simulink model "Lab_7_task_1_4"  (R2020b)
settings: Solver=ode113  StartTime=0.0  StopTime=T  RelTol=1e-13
values from neighbouring files (symbols this model uses):
  a = 8.6251e+06    (= 8625100)    [Quaternions_method_parameters.m]    (also in car2kep.m = -(mu/(2*E)))
  e = norm(e)    [Lab_7_task_1_4_parameters.m]    (also in Lab_7_task_5_parameters.m; Quaternions_method_parameters.m = 0.1195; car2kep.m = 1/mu * [((v_norm)^2 - (mu/r_norm)).*r - (dot(r, v).*v)])
  G = 6.67259e-11    [Lab_7_task_1_4_parameters.m]    (also in Lab_7_task_5_parameters.m; Quaternions_method_parameters.m)
  i = acos(h_z/h_norm)    [car2kep.m]
  I_x = 0.04    [Lab_7_task_1_4_parameters.m]    (also in Lab_7_task_5_parameters.m)
  I_y = 0.06    [Lab_7_task_1_4_parameters.m]    (also in Lab_7_task_5_parameters.m)
  I_z = 0.08    [Lab_7_task_1_4_parameters.m]    (also in Lab_7_task_5_parameters.m)
  m_t = 5.9726*10^24    (= 5.9726e+24)    [Lab_7_task_1_4_parameters.m]    (also in Lab_7_task_5_parameters.m)
  th_0 = 0    [Lab_7_task_1_4_parameters.m]    (also in Lab_7_task_5_parameters.m)
  w_x_0 = 1e-6    (= 1e-06)    [Lab_7_task_1_4_parameters.m]    (also in Lab_7_task_5_parameters.m)
  w_y_0 = 1e-6    (= 1e-06)    [Lab_7_task_1_4_parameters.m]    (also in Lab_7_task_5_parameters.m)
  w_z_0 = n_S    [Lab_7_task_1_4_parameters.m]    (also in Lab_7_task_5_parameters.m)
undefined symbols (not defined in the file or in its folder): magnitude
libraries: robotcorelib x2
settings Model: Creator=39342  LastModifiedBy=39342

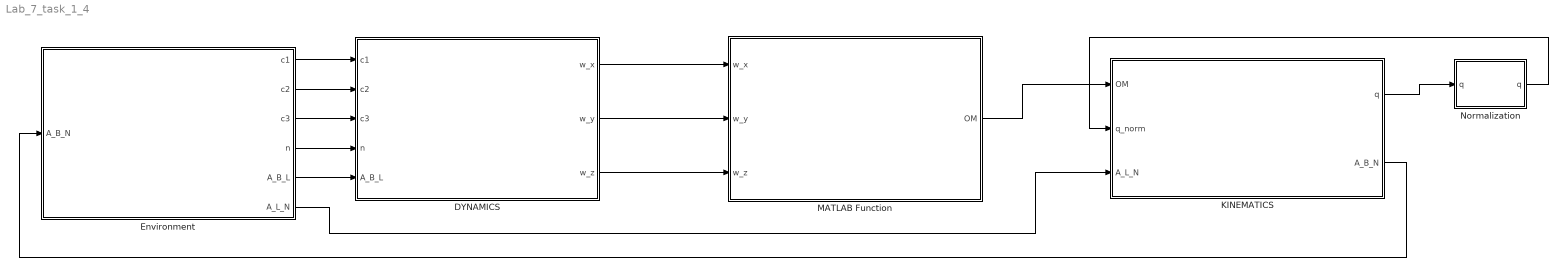
== system Lab_7_task_1_4 ==
  DYNAMICS : Subsystem
  Environment : Subsystem
  KINEMATICS : Subsystem
  MATLAB Function : MATLAB Function  TreatAsAtomicUnit=on
  Normalization : MATLAB Function  TreatAsAtomicUnit=on
  wires:
  Environment/3(c3) -> DYNAMICS/3(c3)
  Environment/1(c1) -> DYNAMICS/1(c1)
  DYNAMICS/1(w_x) -> MATLAB Function/1(w_x)
  Environment/2(c2) -> DYNAMICS/2(c2)
  DYNAMICS/2(w_y) -> MATLAB Function/2(w_y)
  DYNAMICS/3(w_z) -> MATLAB Function/3(w_z)
  Normalization/1(q) -> KINEMATICS/2(q_norm)
  MATLAB Function/1(OM) -> KINEMATICS/1(OM)
  KINEMATICS/1(q) -> Normalization/1("q ")
  KINEMATICS/2(A_B_N) -> Environment/1(A_B_N)
  Environment/4(n) -> DYNAMICS/4(n)
  Environment/5(A_B_L) -> DYNAMICS/5(A_B_L)
  Environment/6(A_L_N) -> KINEMATICS/3(A_L_N)

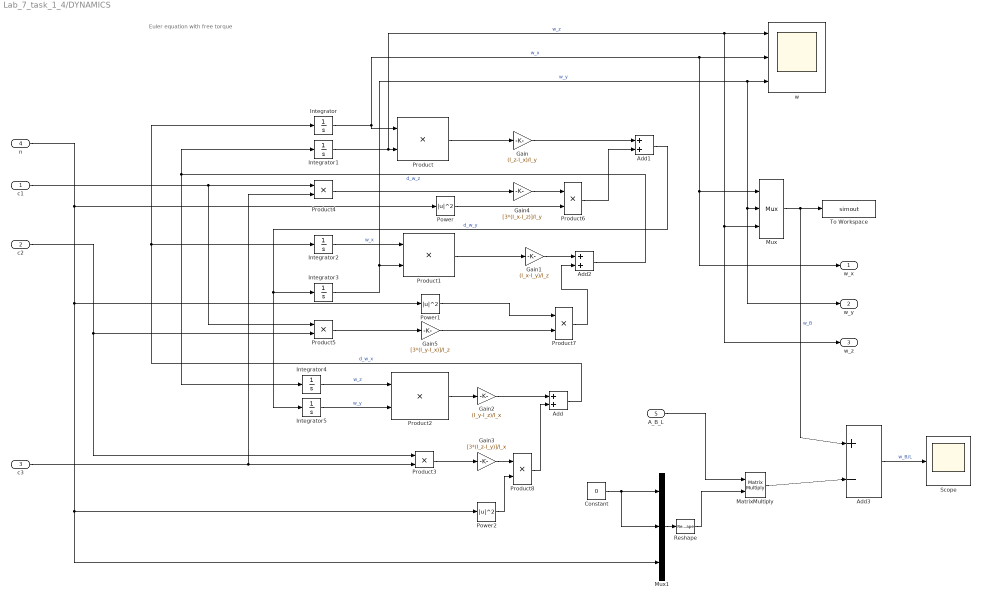
== system Lab_7_task_1_4/DYNAMICS ==
  note: Euler equation with free torque
  c1 : Inport
  c2 : Inport  Port=2
  c3 : Inport  Port=3
  n : Inport  Port=4
  A_B_L : Inport  Port=5
  Add : Sum
  Add1 : Sum
  Add2 : Sum
  Add3 : Sum  Inputs=+|-
  Constant : Constant  Value=0
  Gain : Gain  Gain=(I_z-I_x)/I_y
  Gain1 : Gain  Gain=(I_x-I_y)/I_z
  Gain2 : Gain  Gain=(I_y-I_z)/I_x
  Gain3 : Gain  Gain=[3*(I_z-I_y)]/I_x
  Gain4 : Gain  Gain=[3*(I_x-I_z)]/I_y
  Gain5 : Gain  Gain=[3*(I_y-I_x)]/I_z
  Integrator : Integrator  InitialCondition=w_x_0
  Integrator1 : Integrator  InitialCondition=w_z_0
  Integrator2 : Integrator  InitialCondition=w_x_0
  Integrator3 : Integrator  InitialCondition=w_y_0
  Integrator4 : Integrator  InitialCondition=w_z_0
  Integrator5 : Integrator  InitialCondition=w_y_0
  MatrixMultiply : Product  Multiplication=Matrix(*)
  Mux : Mux  Inputs=3
  Mux1 : Mux  Inputs=3
  Power : Math  Operator=magnitude^2  SaturateOnIntegerOverflow=on
  Power1 : Math  Operator=magnitude^2  SaturateOnIntegerOverflow=on
  Power2 : Math  Operator=magnitude^2  SaturateOnIntegerOverflow=on
  Product{,1..8} (9 alike) : Product
  Reshape : Reshape  OutputDimensionality=Column vector (2-D)
  Scope : Scope
  To Workspace : ToWorkspace  VariableName=simout  SaveFormat=Timeseries  SampleTime=-1
  w : Scope  NumInputPorts=3
  w_x : Outport
  w_y : Outport  Port=2
  w_z : Outport  Port=3
  wires:
  Product1/1 -> Gain1/1
  Integrator/1 -> Product/1, w_x/1, Mux/1, w/2  "w_x"
  Integrator2/1 -> Product1/1  "w_x"
  Mux/1 -> To Workspace/1, Add3/1  "w_B"
  Integrator1/1 -> w/1, w_z/1, Mux/3, Product/2  "w_z"
  Integrator5/1 -> Product2/2  "w_y"
  Integrator4/1 -> Product2/1  "w_z"
  Integrator3/1 -> Product1/2, w/3, w_y/1, Mux/2  "w_y"
  Product/1 -> Gain/1
  Product2/1 -> Gain2/1
  Gain2/1 -> Add/1
  c3/1 -> Product3/2, Product4/2
  c2/1 -> Product5/2, Product3/1
  Product3/1 -> Gain3/1
  Add/1 -> Integrator/1, Integrator2/1  "d_w_x"
  c1/1 -> Product5/1, Product4/1
  Product4/1 -> Gain4/1
  Gain/1 -> Add1/1
  Add1/1 -> Integrator5/1, Integrator3/1  "d_w_y"
  Product5/1 -> Gain5/1
  Gain1/1 -> Add2/1
  Add2/1 -> Integrator4/1, Integrator1/1  "d_w_z"
  Gain4/1 -> Product6/1
  n/1 -> Mux1/3, Power2/1, Power1/1, Power/1
  Power/1 -> Product6/2
  Product6/1 -> Add1/2
  Power1/1 -> Product7/1
  Gain5/1 -> Product7/2
  Product7/1 -> Add2/2
  Power2/1 -> Product8/2
  Gain3/1 -> Product8/1
  Product8/1 -> Add/2
  Constant/1 -> Mux1/2, Mux1/1
  A_B_L/1 -> MatrixMultiply/1
  Mux1/1 -> Reshape/1
  MatrixMultiply/1 -> Add3/2
  Add3/1 -> Scope/1  "w_B/L"
  Reshape/1 -> MatrixMultiply/2

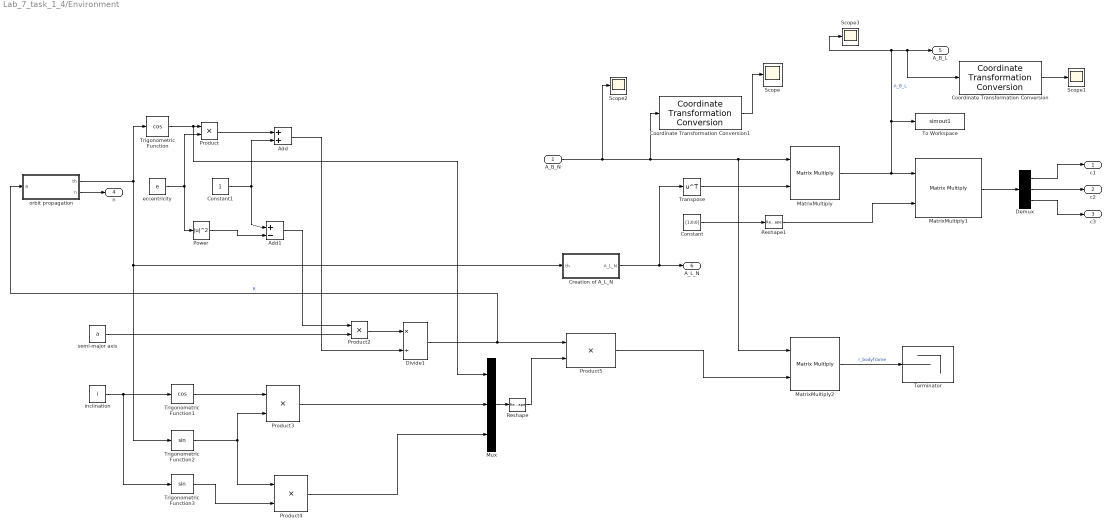
== system Lab_7_task_1_4/Environment ==
  A_B_N : Inport
  Add : Sum
  Add1 : Sum  Inputs=+|-
  Constant : Constant  Value=[1;0;0]
  Constant1 : Constant
  Coordinate Transformation Conversion : robotcorelib/Coordinate Transformation Conversion  InputRepresentation=Rotation Matrix  InputEulerSequence=ZYX  ShowTrVecInputPort=on  OutputRepresentation=Euler Angles  OutputEulerSequence=ZYX  ShowTrVecOutputPort=on  SimulateUsing=Interpreted execution
      settings: SourceProductBaseCode=NV,RO,RR,UV
  Coordinate Transformation Conversion1 : robotcorelib/Coordinate Transformation Conversion  InputRepresentation=Rotation Matrix  InputEulerSequence=ZYX  ShowTrVecInputPort=on  OutputRepresentation=Euler Angles  OutputEulerSequence=ZYX  ShowTrVecOutputPort=on  SimulateUsing=Interpreted execution
      settings: SourceProductBaseCode=NV,RO,RR,UV
  Creation of A_L_N : Subsystem
  Demux : Demux  Outputs=3
  Divide1 : Product  Inputs=*/
  MatrixMultiply : Product  Multiplication=Matrix(*)
  MatrixMultiply1 : Product  Multiplication=Matrix(*)
  MatrixMultiply2 : Product  Multiplication=Matrix(*)
  Mux : Mux  Inputs=3
  Power : Math  Operator=magnitude^2  SaturateOnIntegerOverflow=on
  Product{,2..5} (5 alike) : Product
  Reshape : Reshape  OutputDimensionality=Column vector (2-D)
  Reshape1 : Reshape  OutputDimensionality=Column vector (2-D)
  Scope{,1..3} (4 alike) : Scope
  Terminator : Terminator
  To Workspace : ToWorkspace  VariableName=simout1  SaveFormat=Timeseries  SampleTime=-1
  Transpose : Math  Operator=transpose  SaturateOnIntegerOverflow=on
  Trigonometric Function : Trigonometry  Operator=cos
  Trigonometric Function1 : Trigonometry  Operator=cos
  Trigonometric Function2 : Trigonometry
  Trigonometric Function3 : Trigonometry
  eccentricity : Constant  Value=e
  inclination : Constant  Value=i
  orbit propagation : Subsystem
  semi-major axis : Constant  Value=a
  c1 : Outport
  c2 : Outport  Port=2
  c3 : Outport  Port=3
  n : Outport  Port=4
  A_B_L : Outport  Port=5
  A_L_N : Outport  Port=6
  wires:
  A_B_N/1 -> Scope2/1, Coordinate Transformation Conversion1/1, MatrixMultiply/1, MatrixMultiply2/1
  MatrixMultiply/1 -> Scope3/1, Coordinate Transformation Conversion/1, A_B_L/1, To Workspace/1, MatrixMultiply1/1  "A_B_L"
  Constant/1 -> Reshape1/1
  Demux/1 -> c1/1
  Demux/2 -> c2/1
  Demux/3 -> c3/1
  MatrixMultiply1/1 -> Demux/1
  Trigonometric Function/1 -> Mux/1, Product/1
  Creation of A_L_N/1(A_L_N) -> Transpose/1, A_L_N/1
  Transpose/1 -> MatrixMultiply/2
  semi-major axis/1 -> Product2/2
  Product2/1 -> Divide1/1
  inclination/1 -> Trigonometric Function3/1, Trigonometric Function1/1
  Trigonometric Function1/1 -> Product3/1
  Trigonometric Function2/1 -> Product4/1, Product3/2
  Product3/1 -> Mux/2
  Trigonometric Function3/1 -> Product4/2
  Product4/1 -> Mux/3
  Divide1/1 -> orbit propagation/1(R), Product5/1  "R"
  Mux/1 -> Reshape/1
  Product5/1 -> MatrixMultiply2/2
  MatrixMultiply2/1 -> Terminator/1  "r_bodyframe"
  orbit propagation/1(th) -> Trigonometric Function2/1, Creation of A_L_N/1(th), Trigonometric Function/1
  eccentricity/1 -> Power/1, Product/2
  Product/1 -> Add/1
  Constant1/1 -> Add1/1, Add/2
  Add/1 -> Divide1/2
  Power/1 -> Add1/2
  Add1/1 -> Product2/1
  orbit propagation/2(n) -> n/1
  Coordinate Transformation Conversion/1 -> Scope1/1
  Coordinate Transformation Conversion1/1 -> Scope/1
  Reshape/1 -> Product5/2
  Reshape1/1 -> MatrixMultiply1/2

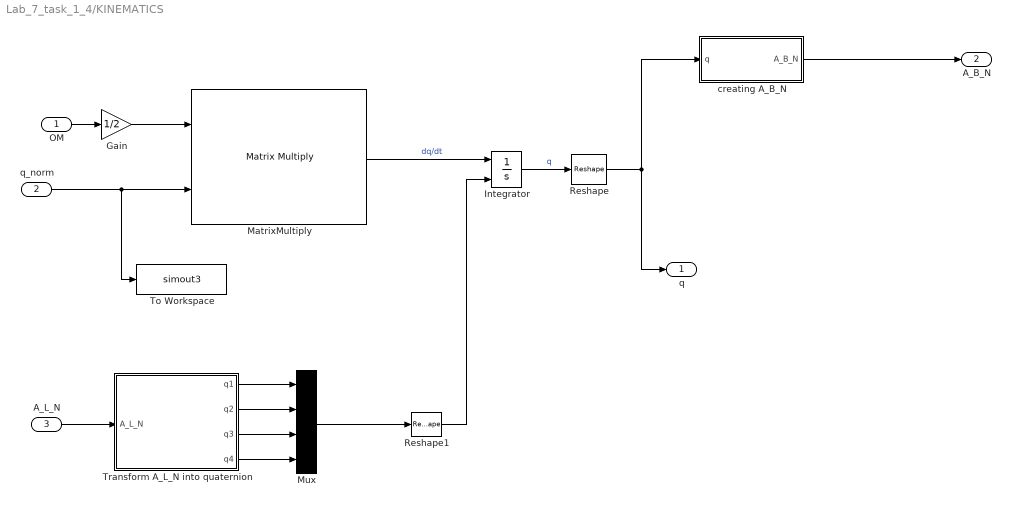
== system Lab_7_task_1_4/KINEMATICS ==
  OM : Inport
  q_norm : Inport  Port=2
  A_L_N : Inport  Port=3
  Gain : Gain  Gain=1/2
  Integrator : Integrator  InitialConditionSource=external  InitialCondition=[0; 0;0;1]
  MatrixMultiply : Product  Multiplication=Matrix(*)
  Mux : Mux
  Reshape : Reshape  OutputDimensionality=Column vector (2-D)
  Reshape1 : Reshape  OutputDimensionality=Column vector (2-D)
  To Workspace : ToWorkspace  VariableName=simout3  SaveFormat=Timeseries  SampleTime=-1
  Transform A_L_N into quaternion : Subsystem
  creating A_B_N : Subsystem
  q : Outport
  A_B_N : Outport  Port=2
  wires:
  MatrixMultiply/1 -> Integrator/1  "dq/dt"
  OM/1 -> Gain/1
  Gain/1 -> MatrixMultiply/1
  q_norm/1 -> To Workspace/1, MatrixMultiply/2
  creating A_B_N/1(A_B_N) -> A_B_N/1
  Integrator/1 -> Reshape/1  "q"
  Reshape/1 -> creating A_B_N/1(q), q/1
  A_L_N/1 -> Transform A_L_N into quaternion/1(A_L_N)
  Transform A_L_N into quaternion/1(q1) -> Mux/1
  Transform A_L_N into quaternion/2(q2) -> Mux/2
  Transform A_L_N into quaternion/3(q3) -> Mux/3
  Transform A_L_N into quaternion/4(q4) -> Mux/4
  Mux/1 -> Reshape1/1
  Reshape1/1 -> Integrator/2

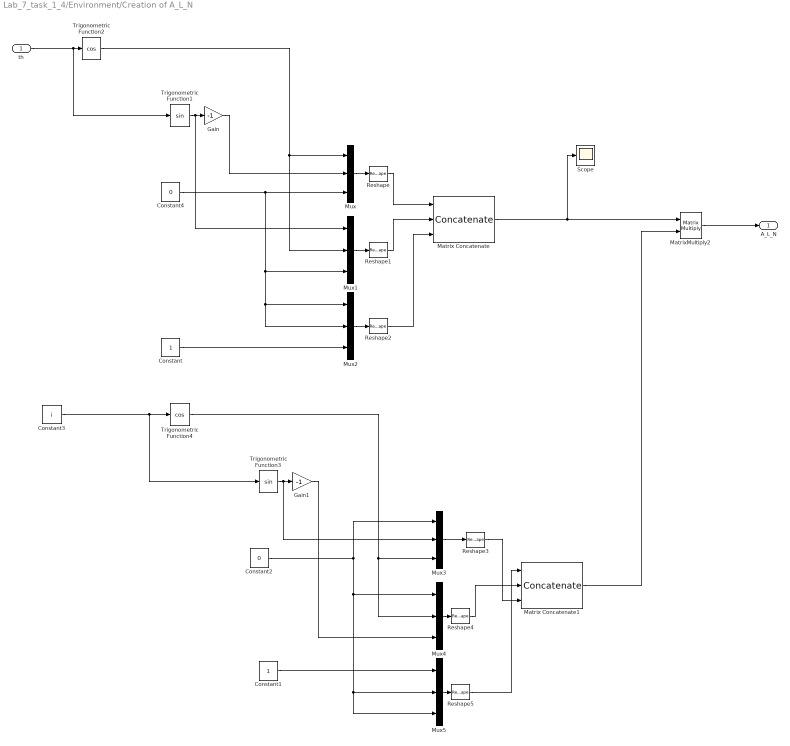
== system Lab_7_task_1_4/Environment/Creation of A_L_N ==
  th : Inport
  Constant : Constant
  Constant1 : Constant
  Constant2 : Constant  Value=0
  Constant3 : Constant  Value=i
  Constant4 : Constant  Value=0
  Gain : Gain  Gain=-1
  Gain1 : Gain  Gain=-1
  Matrix Concatenate : Concatenate  NumInputs=3  Mode=Multidimensional array  ConcatenateDimension=2
  Matrix Concatenate1 : Concatenate  NumInputs=3  Mode=Multidimensional array  ConcatenateDimension=2
  MatrixMultiply2 : Product  Multiplication=Matrix(*)
  Mux{,1..5} (6 alike) : Mux  Inputs=3
  Reshape{,1..5} (6 alike) : Reshape  OutputDimensionality=Column vector (2-D)
  Scope : Scope
  Trigonometric Function1 : Trigonometry
  Trigonometric Function2 : Trigonometry  Operator=cos
  Trigonometric Function3 : Trigonometry
  Trigonometric Function4 : Trigonometry  Operator=cos
  A_L_N : Outport
  wires:
  Mux2/1 -> Reshape2/1
  Gain/1 -> Mux/2
  Trigonometric Function1/1 -> Mux1/1, Gain/1
  Matrix Concatenate/1 -> Scope/1, MatrixMultiply2/1
  Mux1/1 -> Reshape1/1
  Constant4/1 -> Mux2/2, Mux2/1, Mux1/3, Mux/3
  Mux/1 -> Reshape/1
  th/1 -> Trigonometric Function1/1, Trigonometric Function2/1
  Trigonometric Function2/1 -> Mux1/2, Mux/1
  Constant/1 -> Mux2/3
  Trigonometric Function4/1 -> Mux3/3, Mux4/2
  Constant3/1 -> Trigonometric Function3/1, Trigonometric Function4/1
  Trigonometric Function3/1 -> Mux3/2, Gain1/1
  Gain1/1 -> Mux4/3
  Constant2/1 -> Mux3/1, Mux4/1, Mux5/3, Mux5/2
  Constant1/1 -> Mux5/1
  Mux3/1 -> Reshape3/1
  Matrix Concatenate1/1 -> MatrixMultiply2/2
  MatrixMultiply2/1 -> A_L_N/1
  Reshape/1 -> Matrix Concatenate/1
  Reshape1/1 -> Matrix Concatenate/2
  Reshape2/1 -> Matrix Concatenate/3
  Reshape3/1 -> Matrix Concatenate1/3
  Mux4/1 -> Reshape4/1
  Reshape4/1 -> Matrix Concatenate1/2
  Mux5/1 -> Reshape5/1
  Reshape5/1 -> Matrix Concatenate1/1

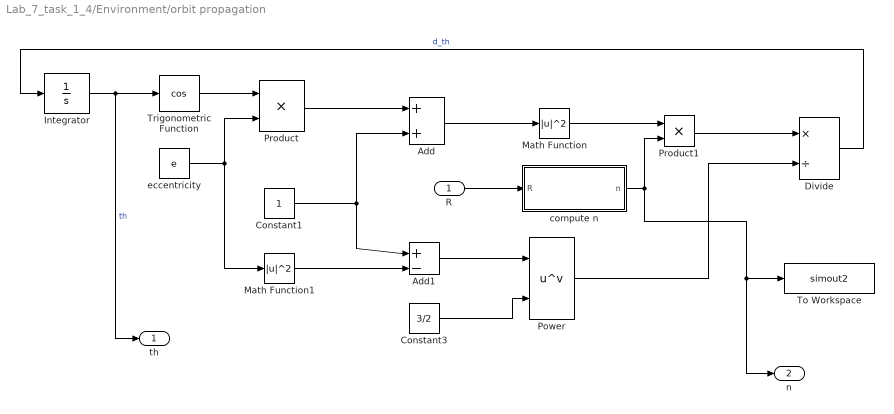
== system Lab_7_task_1_4/Environment/orbit propagation ==
  R : Inport
  Add : Sum
  Add1 : Sum  Inputs=+|-
  Constant1 : Constant
  Constant3 : Constant  Value=3/2
  Divide : Product  Inputs=*/
  Integrator : Integrator  InitialCondition=th_0
  Math Function : Math  Operator=magnitude^2  SaturateOnIntegerOverflow=on
  Math Function1 : Math  Operator=magnitude^2  SaturateOnIntegerOverflow=on
  Power : Math  Operator=pow  SaturateOnIntegerOverflow=on
  Product : Product
  Product1 : Product
  To Workspace : ToWorkspace  VariableName=simout2  SaveFormat=Timeseries  SampleTime=-1
  Trigonometric Function : Trigonometry  Operator=cos
  compute n : Subsystem
  eccentricity : Constant  Value=e
  th : Outport
  n : Outport  Port=2
  wires:
  Math Function1/1 -> Add1/2
  Trigonometric Function/1 -> Product/1
  Divide/1 -> Integrator/1  "d_th"
  Add1/1 -> Power/1
  Power/1 -> Divide/2
  Product/1 -> Add/1
  Product1/1 -> Divide/1
  Add/1 -> Math Function/1
  Integrator/1 -> Trigonometric Function/1, th/1  "th"
  eccentricity/1 -> Product/2, Math Function1/1
  Math Function/1 -> Product1/1
  Constant1/1 -> Add1/1, Add/2
  Constant3/1 -> Power/2
  R/1 -> compute n/1(R)
  compute n/1(n) -> n/1, To Workspace/1, Product1/2

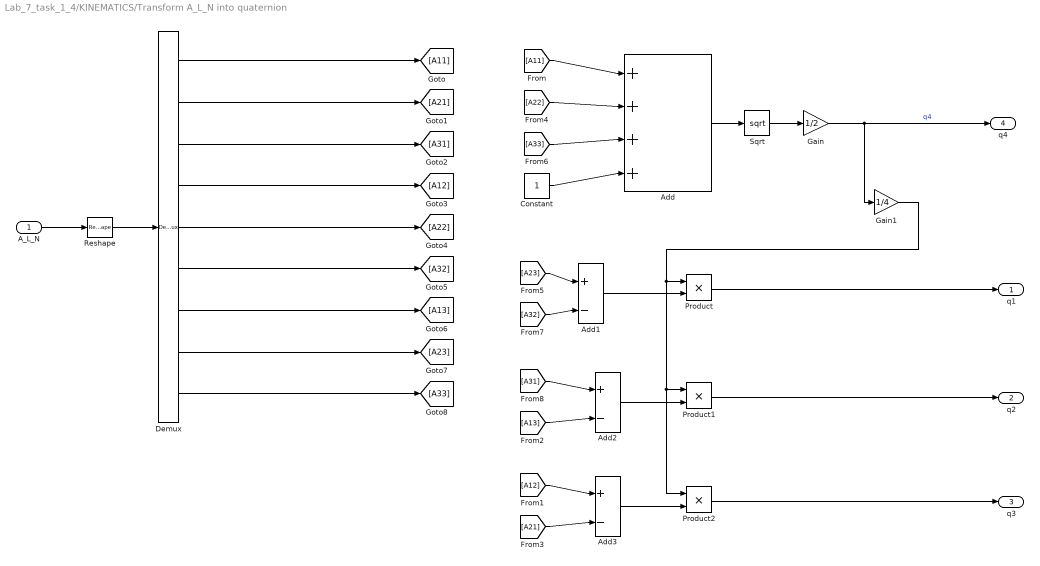
== system Lab_7_task_1_4/KINEMATICS/Transform A_L_N into quaternion ==
  A_L_N : Inport
  Add : Sum  Inputs=+|+|+|+
  Add1 : Sum  Inputs=+|-
  Add2 : Sum  Inputs=+|-
  Add3 : Sum  Inputs=+|-
  Constant : Constant
  Demux : Demux  Outputs=9
  Gain : Gain  Gain=1/2
  Gain1 : Gain  Gain=1/4
  Product : Product
  Product1 : Product
  Product2 : Product
  Reshape : Reshape  OutputDimensionality=Column vector (2-D)
  Sqrt : Sqrt  SaturateOnIntegerOverflow=on
  q1 : Outport
  q2 : Outport  Port=2
  q3 : Outport  Port=3
  q4 : Outport  Port=4
  wires:
  Constant/1 -> Add/4
  [A22] -> Add/2
  [A11] -> Add/1
  [A33] -> Add/3
  Add/1 -> Sqrt/1
  Sqrt/1 -> Gain/1
  Gain/1 -> Gain1/1, q4/1  "q4"
  [A23] -> Add1/1
  [A32] -> Add1/2
  Add1/1 -> Product/2
  Gain1/1 -> Product2/1, Product1/1, Product/1
  Product/1 -> q1/1
  [A31] -> Add2/1
  [A13] -> Add2/2
  Add2/1 -> Product1/2
  Product1/1 -> q2/1
  [A12] -> Add3/1
  [A21] -> Add3/2
  Add3/1 -> Product2/2
  Product2/1 -> q3/1
  A_L_N/1 -> Reshape/1
  Reshape/1 -> Demux/1
  Demux/1 -> [A11]
  Demux/2 -> [A21]
  Demux/3 -> [A31]
  Demux/4 -> [A12]
  Demux/5 -> [A22]
  Demux/6 -> [A32]
  Demux/7 -> [A13]
  Demux/8 -> [A23]
  Demux/9 -> [A33]

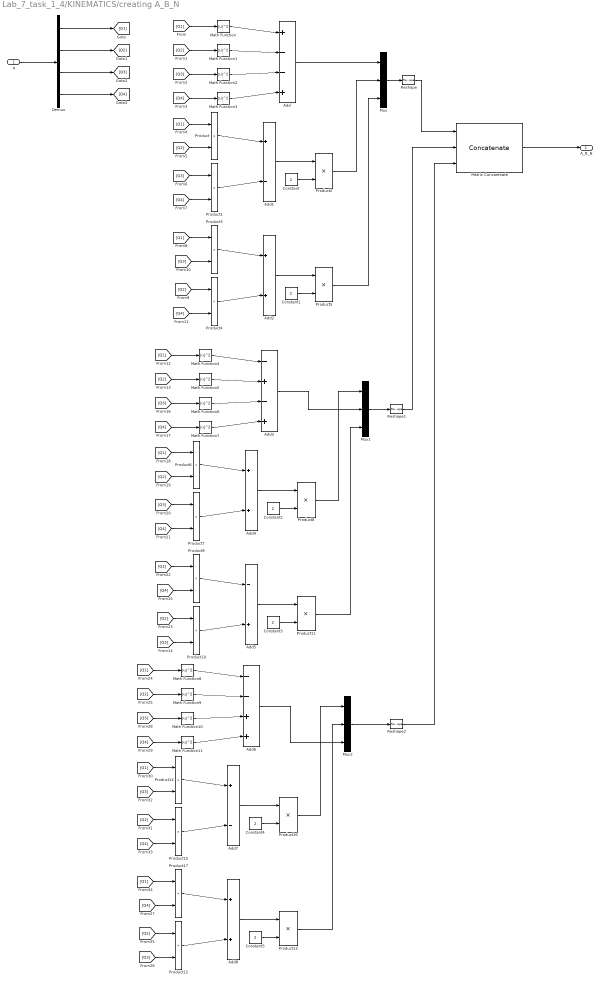
== system Lab_7_task_1_4/KINEMATICS/creating A_B_N ==
  q : Inport
  Add : Sum  Inputs=+|-|-|+
  Add1 : Sum  Inputs=+|-
  Add2 : Sum  Inputs=+|+
  Add3 : Sum  Inputs=-|+|-|+
  Add4 : Sum  Inputs=+|+
  Add5 : Sum  Inputs=-|+
  Add6 : Sum  Inputs=-|-|+|+
  Add7 : Sum  Inputs=+|-
  Add8 : Sum  Inputs=+|+
  Constant{,1..5} (6 alike) : Constant  Value=2
  Demux : Demux
  Math Function{,1..11} (12 alike) : Math  Operator=magnitude^2  SaturateOnIntegerOverflow=on
  Matrix Concatenate : Concatenate  NumInputs=3  Mode=Multidimensional array  ConcatenateDimension=2
  Mux : Mux  Inputs=3
  Mux1 : Mux  Inputs=3
  Mux2 : Mux  Inputs=3
  Product{,1..17} (18 alike) : Product
  Reshape : Reshape  OutputDimensionality=Column vector (2-D)
  Reshape1 : Reshape  OutputDimensionality=Column vector (2-D)
  Reshape2 : Reshape  OutputDimensionality=Column vector (2-D)
  A_B_N : Outport
  wires:
  q/1 -> Demux/1
  Demux/1 -> [Q1]
  Demux/2 -> [Q2]
  Demux/3 -> [Q3]
  Demux/4 -> [Q4]
  [Q1] -> Math Function/1
  Math Function/1 -> Add/1
  [Q2] -> Math Function1/1
  Math Function1/1 -> Add/2
  [Q4] -> Math Function3/1
  Math Function3/1 -> Add/4
  [Q3] -> Math Function2/1
  Math Function2/1 -> Add/3
  [Q2] -> Product/2
  [Q1] -> Product/1
  [Q3] -> Product1/1
  [Q4] -> Product1/2
  Product/1 -> Add1/1
  Product1/1 -> Add1/2
  Add1/1 -> Product2/1
  Constant/1 -> Product2/2
  Product3/1 -> Add2/1
  Constant1/1 -> Product5/2
  [Q4] -> Product4/2
  Add2/1 -> Product5/1
  Product4/1 -> Add2/2
  [Q1] -> Product3/1
  [Q3] -> Product3/2
  [Q2] -> Product4/1
  Add/1 -> Mux/1
  Product2/1 -> Mux/2
  Product5/1 -> Mux/3
  [Q2] -> Product10/1
  Product10/1 -> Add5/2
  Add5/1 -> Product11/1
  Product9/1 -> Add5/1
  Constant2/1 -> Product8/2
  [Q4] -> Product7/2
  [Q1] -> Product6/1
  Constant3/1 -> Product11/2
  [Q3] -> Product7/1
  Add4/1 -> Product8/1
  [Q1] -> Math Function4/1
  Product6/1 -> Add4/1
  Product7/1 -> Add4/2
  Math Function5/1 -> Add3/2
  [Q1] -> Product9/1
  Math Function7/1 -> Add3/4
  [Q2] -> Product6/2
  Product8/1 -> Mux1/1
  [Q3] -> Math Function6/1
  [Q4] -> Math Function7/1
  Math Function6/1 -> Add3/3
  [Q2] -> Math Function5/1
  Math Function4/1 -> Add3/1
  Add3/1 -> Mux1/2
  Product11/1 -> Mux1/3
  [Q4] -> Product9/2
  [Q3] -> Product10/2
  [Q4] -> Math Function11/1
  [Q2] -> Math Function9/1
  Math Function10/1 -> Add6/3
  Math Function11/1 -> Add6/4
  Math Function9/1 -> Add6/2
  [Q1] -> Product17/1
  Product15/1 -> Add7/2
  Math Function8/1 -> Add6/1
  [Q1] -> Math Function8/1
  Add7/1 -> Product16/1
  Constant4/1 -> Product16/2
  Product17/1 -> Add8/1
  [Q4] -> Product15/2
  [Q1] -> Product14/1
  Constant5/1 -> Product13/2
  Product12/1 -> Add8/2
  Add8/1 -> Product13/1
  [Q4] -> Product17/2
  Product14/1 -> Add7/1
  [Q3] -> Math Function10/1
  [Q2] -> Product12/1
  [Q3] -> Product12/2
  [Q3] -> Product14/2
  [Q2] -> Product15/1
  Product16/1 -> Mux2/1
  Product13/1 -> Mux2/2
  Add6/1 -> Mux2/3
  Mux/1 -> Reshape/1
  Mux1/1 -> Reshape1/1
  Mux2/1 -> Reshape2/1
  Matrix Concatenate/1 -> A_B_N/1
  Reshape/1 -> Matrix Concatenate/1
  Reshape1/1 -> Matrix Concatenate/2
  Reshape2/1 -> Matrix Concatenate/3

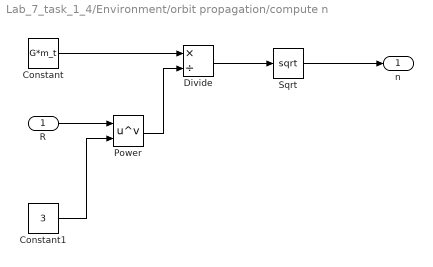
== system Lab_7_task_1_4/Environment/orbit propagation/compute n ==
  R : Inport
  Constant : Constant  Value=G*m_t
  Constant1 : Constant  Value=3
  Divide : Product  Inputs=*/
  Power : Math  Operator=pow  SaturateOnIntegerOverflow=on
  Sqrt : Sqrt  SaturateOnIntegerOverflow=on
  n : Outport
  wires:
  R/1 -> Power/1
  Constant1/1 -> Power/2
  Constant/1 -> Divide/1
  Power/1 -> Divide/2
  Divide/1 -> Sqrt/1
  Sqrt/1 -> n/1

== matlab function Lab_7_task_1_4/Normalization ==
  data: q input; q output
function q = fcn(q)


q = q/norm(q);

end

== matlab function Lab_7_task_1_4/MATLAB Function ==
  data: w_x input; w_y input; w_z input; OM output
function OM = fcn(w_x, w_y, w_z)

OM = [0, w_z, -w_y, w_x; -w_z, 0, w_x, w_y; w_y, -w_x, 0, w_z; -w_x, -w_y, -w_z, 0];
end
